simulink model "try_slp"  (R2021a)
settings: Solver=ode1  StartTime=0.0  StopTime=20.0  FixedStep=0.001  RelTol=1e-3
libraries: simulink x4
settings Model: Creator=tejal  LastModifiedBy=tejal

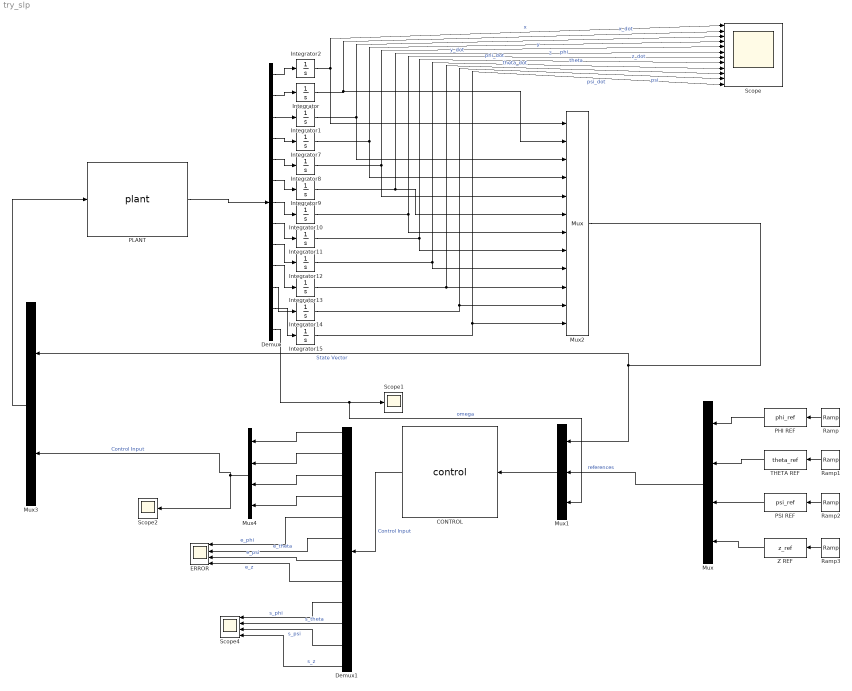
== system try_slp ==
  CONTROL : MATLABFcn  MATLABFcn=control  OutputDimensions=12
  Demux : Demux  Outputs=13
  Demux1 : Demux  Outputs=12
  ERROR : Scope  NumInputPorts=4
  Integrator{,1..2,7..15} (12 alike) : Integrator
  Mux : Mux
  Mux1 : Mux  Inputs=3
  Mux2 : Mux  Inputs=12
  Mux3 : Mux  Inputs=2
  Mux4 : Mux
  PHI REF : MATLABFcn  MATLABFcn=phi_ref  OutputDimensions=3
  PLANT : MATLABFcn  MATLABFcn=plant  OutputDimensions=13
  PSI REF : MATLABFcn  MATLABFcn=psi_ref  OutputDimensions=3
  Ramp : simulink/Sources/Ramp  slope=0.01  start=0  InitialOutput=0
  Ramp1 : simulink/Sources/Ramp  slope=1  start=0  InitialOutput=0
  Ramp2 : simulink/Sources/Ramp  slope=1  start=0  InitialOutput=0
  Ramp3 : simulink/Sources/Ramp  slope=1  start=0  InitialOutput=0
  Scope : Scope  NumInputPorts=12
  Scope1 : Scope
  Scope2 : Scope
  Scope4 : Scope  NumInputPorts=4
  THETA REF : MATLABFcn  MATLABFcn=theta_ref  OutputDimensions=3
  Z REF : MATLABFcn  MATLABFcn=z_ref  OutputDimensions=3
  wires:
  Ramp/1 -> PHI REF/1
  Ramp1/1 -> THETA REF/1
  Ramp2/1 -> PSI REF/1
  Ramp3/1 -> Z REF/1
  PHI REF/1 -> Mux/1
  THETA REF/1 -> Mux/2
  PLANT/1 -> Demux/1
  Demux/2 -> Integrator/1
  Demux/12 -> Integrator15/1
  Demux/11 -> Integrator14/1
  Demux/10 -> Integrator13/1
  Demux/9 -> Integrator12/1
  Demux/8 -> Integrator11/1
  Demux/7 -> Integrator10/1
  Demux/6 -> Integrator9/1
  Demux/5 -> Integrator8/1
  Demux/4 -> Integrator7/1
  Demux/3 -> Integrator1/1
  Integrator/1 -> Mux2/2, Scope/2  "x_dot"
  Integrator1/1 -> Mux2/3, Scope/3  "y"
  Integrator7/1 -> Scope/4, Mux2/4  "y_dot"
  Integrator8/1 -> Mux2/5, Scope/5  "z"
  Integrator9/1 -> Mux2/6, Scope/6  "z_dot"
  Integrator10/1 -> Scope/7, Mux2/7  "phi"
  Integrator11/1 -> Mux2/8, Scope/8  "phi_dot"
  Integrator12/1 -> Mux2/9, Scope/9  "theta"
  Integrator13/1 -> Mux2/10, Scope/10  "theta_dot"
  Integrator14/1 -> Mux2/11, Scope/11  "psi"
  Integrator15/1 -> Mux2/12, Scope/12  "psi_dot"
  Demux/1 -> Integrator2/1
  Integrator2/1 -> Scope/1, Mux2/1  "x"
  Mux/1 -> Mux1/2  "references"
  Mux1/1 -> CONTROL/1
  Mux2/1 -> Mux3/1, Mux1/1  "State Vector"
  Mux4/1 -> Scope2/1, Mux3/2  "Control Input"
  Mux3/1 -> PLANT/1
  PSI REF/1 -> Mux/3
  Z REF/1 -> Mux/4
  Demux/13 -> Mux1/3, Scope1/1  "omega"
  CONTROL/1 -> Demux1/1  "Control Input"
  Demux1/1 -> Mux4/1
  Demux1/2 -> Mux4/2
  Demux1/3 -> Mux4/3
  Demux1/4 -> Mux4/4
  Demux1/5 -> ERROR/1  "e_phi"
  Demux1/6 -> ERROR/2  "e_theta"
  Demux1/7 -> ERROR/3  "e_psi"
  Demux1/8 -> ERROR/4  "e_z"
  Demux1/9 -> Scope4/1  "s_phi"
  Demux1/10 -> Scope4/2  "s_theta"
  Demux1/11 -> Scope4/3  "s_psi"
  Demux1/12 -> Scope4/4  "s_z"
